simulink model "data_acquisition_model"  (R2018b)
settings: Solver=VariableStepAuto  StartTime=0.0  StopTime=10.0  RelTol=1e-3
undefined symbols (not defined in the file or in its folder): sigbuilder_block
libraries: fl_lib x10, nesl_utility x5
settings Model: Creator=andrey.yershov  LastModifiedBy=andrey.yershov

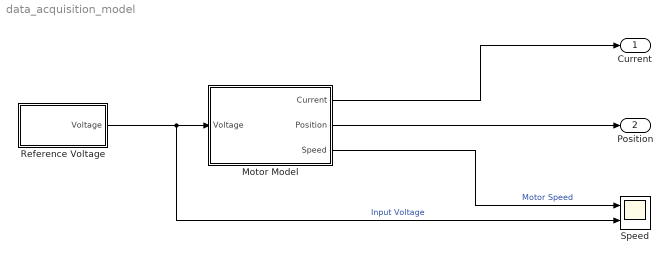
== system data_acquisition_model ==
  Motor Model : Subsystem
  Reference Voltage : Subsystem  Tag=STV Subsys  LoadFcn=sigbuilder_block('load');  StartFcn=sigbuilder_block('start');  StopFcn=sigbuilder_block('stop');  ClipboardFcn=sigbuilder_block('clipboard');  mask(Sigbuilder block){tuvar=[0:10]}
      mask help: Sigbuilder GUI
      mask init:
      | if ~strcmp(get_param(bdroot(gcbh),'SimulationStatus'),'stopped') tuvar = sigbuilder_block('maskInit'); end
      settings: CopyFcn=sigbuilder_block('copy');  DeleteFcn=sigbuilder_block('delete');  ModelCloseFcn=sigbuilder_block('modelClose');  PreSaveFcn=sigbuilder_block('preSave');  PauseFcn=sigbuilder_block('pause')  ContinueFcn=sigbuilder_block('continue')  NameChangeFcn=sigbuilder_block('namechange');  OpenFcn=sigbuilder_block('open',[6 60.75 402 361.5 ]);  CloseFcn=sigbuilder_block('close');
      mask Display: plot(0, 0, 100, 100,[2, 2, 32, 32, 2], [68, 8, 8, 68, 68],[32, 2], [38, 38], [32, 19, 2],[53, 60, 44], [32, 17, 17, 2],[16, 16, 31, 31]);txt = getActiveGroup(gcbh);text(2, 100, txt,'verticalAlignment', 'top');
  Speed : Scope  NumInputPorts=2
  Current : Outport
  Position : Outport  Port=2
  wires:
  Reference Voltage/1(Voltage) -> Speed/2, Motor Model/1(Voltage)  "Input Voltage"
  Motor Model/1(Current) -> Current/1
  Motor Model/2(Position) -> Position/1
  Motor Model/3(Speed) -> Speed/1  "Motor Speed"

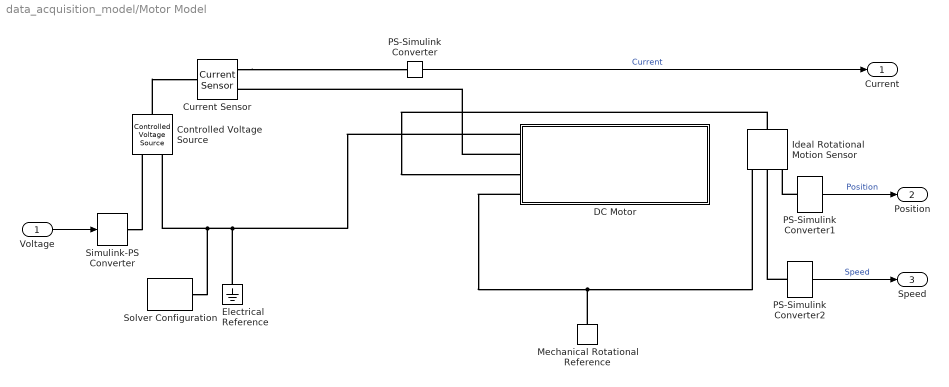
== system data_acquisition_model/Motor Model ==
  Voltage : Inport
  Controlled Voltage Source : fl_lib/Electrical/Electrical Sources/Controlled Voltage Source
  Current Sensor : fl_lib/Electrical/Electrical Sensors/Current Sensor
  DC Motor : Subsystem
  Electrical Reference : fl_lib/Electrical/Electrical Elements/Electrical Reference
  Ideal Rotational Motion Sensor : fl_lib/Mechanical/Mechanical Sensors/Ideal Rotational Motion Sensor  offset=0 rad
  Mechanical Rotational Reference : fl_lib/Mechanical/Rotational Elements/Mechanical Rotational Reference
  PS-Simulink Converter : nesl_utility/PS-Simulink Converter  PhysicalDomain=network_engine_domain  SubClassName=ps_output  LeftPortType=input  RightPortType=output  PseudoPeriodic=off  Frequencies=[]  Unit=1  AffineConversion=off
  PS-Simulink Converter1 : nesl_utility/PS-Simulink Converter  PhysicalDomain=network_engine_domain  SubClassName=ps_output  LeftPortType=input  RightPortType=output  PseudoPeriodic=off  Frequencies=[]  Unit=1  AffineConversion=off
  PS-Simulink Converter2 : nesl_utility/PS-Simulink Converter  PhysicalDomain=network_engine_domain  SubClassName=ps_output  LeftPortType=input  RightPortType=output  PseudoPeriodic=off  Frequencies=[]  Unit=1  AffineConversion=off
  Simulink-PS Converter : nesl_utility/Simulink-PS Converter  PhysicalDomain=network_engine_domain  SubClassName=ps_input  LeftPortType=input  RightPortType=output  PseudoPeriodic=off  Frequencies=[]  NoiseDistribution=none  NoiseParameters=[]  Unit=1  AffineConversion=off  FilteringAndDerivatives=provide  SimscapeFilterOrder=1  InputFilterTimeConstant=0.001  UdotUserProvided=0
  Solver Configuration : nesl_utility/Solver Configuration  PhysicalDomain=network_engine_domain  SubClassName=solver  LeftPortType=input  RightPortType=generic  Tones=[]  Harmonics=[]  SimulateNoise=off  Profile=off  UseLocalSampling=off  EnableSwitchedLinearOptims=on  FrequencyDomain=off  UseCCode=off  RelTol=0.001  AbsTol=1e-06  MinStep=1e-09  ToWorkspace=off  RevertToSquareIcSolve=off  NumHomotopyIterations=100  PhasorMode=off  PhasorModeNumHarmonics=1  DoDC=off  ResidualTolerance=1e-09  UseLocalSolver=off  LocalSolverChoice=NE_BACKWARD_EULER_ADVANCER  LocalSolverSampleTime=0.001  DoFixedCost=off  MaxNonlinIter=3  MaxModeIter=2  LinearAlgebra=auto  EquationFormulation=NE_TIME_EF  DelaysMemoryBudget=1024  AutomaticFiltering=on  FilteringTimeConstant=0.001  PartitionStorageMethod=AS_NEEDED  PartitionMemoryBudget=1024
  Current : Outport
  Position : Outport  Port=2
  Speed : Outport  Port=3
  wires:
  PS-Simulink Converter2/1 -> Speed/1  "Speed"
  Voltage/1 -> Simulink-PS Converter/1
  PS-Simulink Converter1/1 -> Position/1  "Position"
  PS-Simulink Converter/1 -> Current/1  "Current"
  connections:
  PS-Simulink Converter2/LConn1 -- Ideal Rotational Motion Sensor/RConn2
  PS-Simulink Converter1/LConn1 -- Ideal Rotational Motion Sensor/RConn3
  DC Motor/LConn1 -- Controlled Voltage Source/RConn2 -- Solver Configuration/RConn1 -- Electrical Reference/LConn1
  Simulink-PS Converter/RConn1 -- Controlled Voltage Source/RConn1
  DC Motor/LConn4 -- Mechanical Rotational Reference/LConn1 -- Ideal Rotational Motion Sensor/RConn1
  Ideal Rotational Motion Sensor/LConn1 -- DC Motor/LConn3
  DC Motor/LConn2 -- Current Sensor/RConn2
  Controlled Voltage Source/LConn1 -- Current Sensor/LConn1
  Current Sensor/RConn1 -- PS-Simulink Converter/LConn1

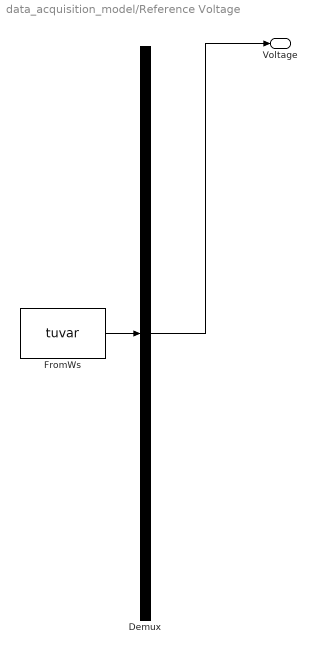
== system data_acquisition_model/Reference Voltage ==
  Demux : Demux  Tag=STV Demux  Outputs=1
  FromWs : FromWorkspace  Tag=STV FromWs  VariableName=tuvar  SampleTime=1/100
      SigBuilderData=|
      | common.afterFinalStr = 'Extrapolate'
      | common.sampleTime = '1/100'
      | dataSet(1).timeRange = [0 10]
      | dataSet(1).name = 'Bounds1_z11'
      | dataSet(2).timeRange = [0 10]
      | dataSet(2).name = 'Bounds5_z4'
      | dataSet(3).timeRange = [0 20]
      | dataSet(3).name = 'Sine3_z1'
      | dataSet(4).timeRange = [0 20]
      | dataSet(4).name = 'Sine5_z2'
      | dataSet(5).timeRange = [0 20]
      | dataSet(5).name = 'Step1_z5'
      | dataSet(6).timeRange = [0 20]
      | dataSet(6).name = 'Step2_z8'
      | dataSet(7).timeRange = [0 10]
      | dataSet(7).name = 'RampSquare_z3'
      | dataSet(8).timeRange = [0 10]
      | dataSet(8).name = 'Steps_z9'
      | dataSet(9).timeRange = [0 10]
      | dataSet(9).name = 'Small Steps_z6'
      | dataSet(10).timeRange = [0 10]
      | dataSet(10).name = 'Square_z10'
      | dataSet(11).timeRange = [0 55]
      | dataSet(11).name = 'DeadZone_z7'
      | sbobj.Groups(1).Name = 'Bounds1_z11'
      | sbobj.Groups(1).Signals.Name = 'Voltage'
      | sbobj.Groups(1).Signals.XData = [0 2.5 2.5 5 5 7.5 7.5 10]
      | sbobj.Groups(1).Signals.YData = [1 1 -1 -1 1 1 -1 -1]
      | sbobj.Groups(2).Name = 'Bounds5_z4'
      | sbobj.Groups(2).Signals.Name = 'Voltage'
      | sbobj.Groups(2).Signals.XData = [0 2.5 2.5 5 5 7.5 7.5 10]
      | sbobj.Groups(2).Signals.YData = [5 5 -5 -5 5 5 -5 -5]
      | sbobj.Groups(3).Name = 'Sine3_z1'
      | sbobj.Groups(3).Signals.Name = 'Voltage'
      | sbobj.Groups(3).Signals.XData = [0 0.01 0.02 0.03 0.04 0.05 0.06 0.07 0.08 0.09 0.1 0.11 ... (2001 elements, 1x2001)]
      | sbobj.Groups(3).Signals.YData = [0 0.0299995000025 0.05999600008 0.0899865006075 0.11996800256 0.149937507812 0.179892019438 0.209828542013 0.239744081908 0.269635647594 0.29950024994 0.329334902512 ... (2001 elements, 1x2001)]
      | sbobj.Groups(3).TimeRange = [0 20]
      | sbobj.Groups(4).Name = 'Sine5_z2'
      | sbobj.Groups(4).Signals.Name = 'Voltage'
      | sbobj.Groups(4).Signals.XData = [0 0.01 0.02 0.03 0.04 0.05 0.06 0.07 0.08 0.09 0.1 0.11 ... (2001 elements, 1x2001)]
      | sbobj.Groups(4).Signals.YData = [0 0.0499991666708 0.0999933334667 0.149977501012 0.199946670933 0.249895846353 0.299820032397 0.349714236688 0.399573469846 0.44939274599 0.499167083234 0.548891504186 ... (2001 elements, 1x2001)]
      | sbobj.Groups(4).TimeRange = [0 20]
      | sbobj.Groups(5).Name = 'Step1_z5'
      | sbobj.Groups(5).Signals.Name = 'Voltage'
      | sbobj.Groups(5).Signals.XData = [0 0.01 0.02 0.03 0.04 0.05 0.06 0.07 0.08 0.09 0.1 0.11 ... (2001 elements, 1x2001)]
      | sbobj.Groups(5).Signals.YData = [0 0 0 0 0 0 0 0 0 0 0 0 ... (2001 elements, 1x2001)]
      | sbobj.Groups(5).TimeRange = [0 20]
      | sbobj.Groups(6).Name = 'Step2_z8'
      | sbobj.Groups(6).Signals.Name = 'Voltage'
      | sbobj.Groups(6).Signals.XData = [0 0.01 0.02 0.03 0.04 0.05 0.06 0.07 0.08 0.09 0.1 0.11 ... (2001 elements, 1x2001)]
      | sbobj.Groups(6).Signals.YData = [0 0 0 0 0 0 0 0 0 0 0 0 ... (2001 elements, 1x2001)]
      | sbobj.Groups(6).TimeRange = [0 20]
      | sbobj.Groups(7).Name = 'RampSquare_z3'
      | sbobj.Groups(7).Signals.Name = 'Voltage'
      | sbobj.Groups(7).Signals.XData = [0 1 1 2 2 3 3 4 4 5 5 6 6 7 7 8 8 9 9 9.8 9.8 10]
      | sbobj.Groups(7).Signals.YData = [0 0.75 0 -0.75 0 1.5 0 -1.5 2 2 -2 -2 3 3 -3 -3 1 1 -1 -1 0 0]
      | sbobj.Groups(8).Name = 'Steps_z9'
      | sbobj.Groups(8).Signals.Name = 'Voltage'
      | sbobj.Groups(8).Signals.XData = [0 1.52 1.52 2.4 2.4 3.66 3.68 4.64 4.64 6.02 6.02 7 7 8.96 8.96 10]
      | sbobj.Groups(8).Signals.YData = [2 2 -3 -3 3 -1 1.95 1.95 -2 -2 0.7 0.7 -1.05 -0.05 0 0]
      | sbobj.Groups(9).Name = 'Small Steps_z6'
      | sbobj.Groups(9).Signals.Name = 'Voltage'
      | sbobj.Groups(9).Signals.XData = [0 0.5 0.5 1.02 1.02 2 2 2.58 2.58 3.78 3.78 4.64 4.64 5.28 5.28 6 6 7 7 9 9 10]
      | sbobj.Groups(9).Signals.YData = [0.4 0.4 0.75 0.75 1.5 3 1.55 1.55 3.55 3.55 -3.05 -3.05 -1 -1 -0.45 -0.45 0.7 0.7 -2.05 -0.05 1 1]
      | sbobj.Groups(10).Name = 'Square_z10'
      | sbobj.Groups(10).Signals.Name = 'Voltage'
      | sbobj.Groups(10).Signals.XData = [0 0.5 0.5 1.02 1.02 1.5 1.5 2 2 2.5 2.5 3 3 4 4 5 5 6 6 7 7 8 8 9 9 9.8 9.8 10]
      | sbobj.Groups(10).Signals.YData = [0.4 0.4 -0.4 -0.4 1 1 -1 -1 1.5 1.5 -1.5 -1.5 2 2 -2 -2 3 3 -3 -3 1.3 1.3 -1.3 -1.3 -4 -4 0 0]
      | sbobj.Groups(11).Name = 'DeadZone_z7'
      | sbobj.Groups(11).Signals.Name = 'Voltage'
      | sbobj.Groups(11).Signals.XData = [0 5 5 10 10 15 15 20 25 30 30 35 40 45 50 50 55]
      | sbobj.Groups(11).Signals.YData = [0 0 0.16 0.16 0.3 0.3 0.7 0.7 -0.205 -0.205 -0.355 -0.35 -0.605 -0.605 0.005 0 0]
      | sbobj.Groups(11).TimeRange = [0 55]
  Voltage : Outport  Tag=STV Outport
  wires:
  FromWs/1 -> Demux/1
  Demux/1 -> Voltage/1

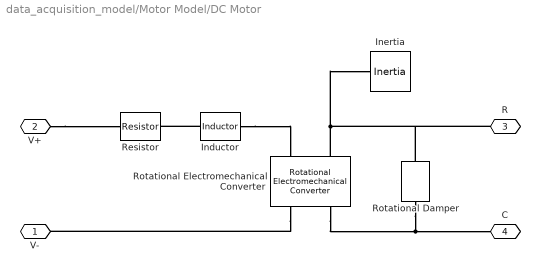
== system data_acquisition_model/Motor Model/DC Motor ==
  Inductor : fl_lib/Electrical/Electrical Elements/Inductor  l=0.5 H  r=0 Ohm  g=1e-9 1/Ohm  i_specify=off  i_priority=None  i=0 A  i_nominal_specify=off  i_nominal_unit=A  i_nominal_value=1  v_specify=off  v_priority=None  v=0 V  v_nominal_specify=off  v_nominal_unit=V  v_nominal_value=1  i_L_specify=off  i_L_priority=High  i_L=0 A  i_L_nominal_specify=off  i_L_nominal_unit=A  i_L_nominal_value=1
  Inertia : fl_lib/Mechanical/Rotational Elements/Inertia  inertia=0.01 kg*m^2  w_specify=off  w_priority=High  w=0 rad/s  w_nominal_specify=off  w_nominal_unit=rad/s  w_nominal_value=1  t_specify=off  t_priority=None  t=0 N*m  t_nominal_specify=off  t_nominal_unit=N*m  t_nominal_value=1
  Resistor : fl_lib/Electrical/Electrical Elements/Resistor  R=1 Ohm  i_specify=off  i_priority=None  i=0 A  i_nominal_specify=off  i_nominal_unit=A  i_nominal_value=1  v_specify=off  v_priority=None  v=0 V  v_nominal_specify=off  v_nominal_unit=V  v_nominal_value=1
  Rotational Electromechanical Converter : fl_lib/Electrical/Electrical Elements/Rotational Electromechanical Converter  K=0.01 V/(rad/s)  i_specify=off  i_priority=None  i=0 A  i_nominal_specify=off  i_nominal_unit=A  i_nominal_value=1  v_specify=off  v_priority=None  v=0 V  v_nominal_specify=off  v_nominal_unit=V  v_nominal_value=1  t_specify=off  t_priority=None  t=0 N*m  t_nominal_specify=off  t_nominal_unit=N*m  t_nominal_value=1  w_specify=off  w_priority=None  w=0 rad/s  w_nominal_specify=off  w_nominal_unit=rad/s  w_nominal_value=1
      settings: SourceProductName=Simscape
  Rotational Damper : fl_lib/Mechanical/Rotational Elements/Rotational Damper  D=0.1 N*m/(rad/s)  w_specify=off  w_priority=None  w=0 rad/s  w_nominal_specify=off  w_nominal_unit=rad/s  w_nominal_value=1  t_specify=off  t_priority=None  t=0 N*m  t_nominal_specify=off  t_nominal_unit=N*m  t_nominal_value=1
  V- : PMIOPort  Side=Left
  V+ : PMIOPort  Port=2  Side=Left
  R : PMIOPort  Port=3  Side=Left
  C : PMIOPort  Port=4  Side=Left
  connections:
  Inductor/RConn1 -- Rotational Electromechanical Converter/LConn1
  Rotational Electromechanical Converter/LConn2 -- R/RConn1 -- Rotational Damper/RConn1 -- Inertia/LConn1
  Rotational Electromechanical Converter/RConn2 -- C/RConn1 -- Rotational Damper/LConn1
  Inductor/LConn1 -- Resistor/RConn1
  Rotational Electromechanical Converter/RConn1 -- V-/RConn1
  V+/RConn1 -- Resistor/LConn1
